simulink model "sistema (1)"  (R2025b)
settings: Solver=ode23t  StartTime=0.0  StopTime=10.0  MaxStep=1e-3  RelTol=1e-3
libraries: slpidlib x1, simulink x1
settings DataIOCC: ReturnWorkspaceOutputs=off  TimeSaveName=t
settings DebuggingCC: AlgebraicLoopMsg=none  ArtificialAlgebraicLoopMsg=none  MaxConsecutiveZCsMsg=none

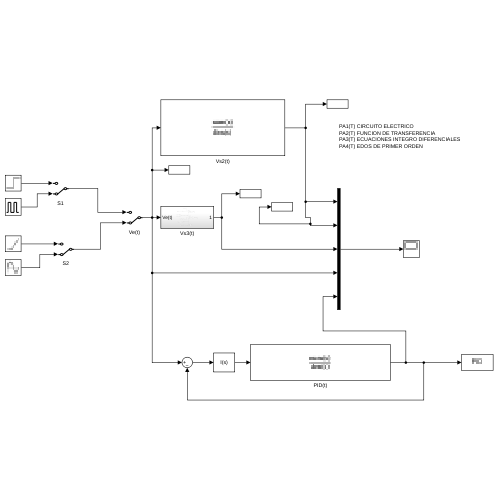
[thumbnail: Simulink's stored preview of the top-level diagram]
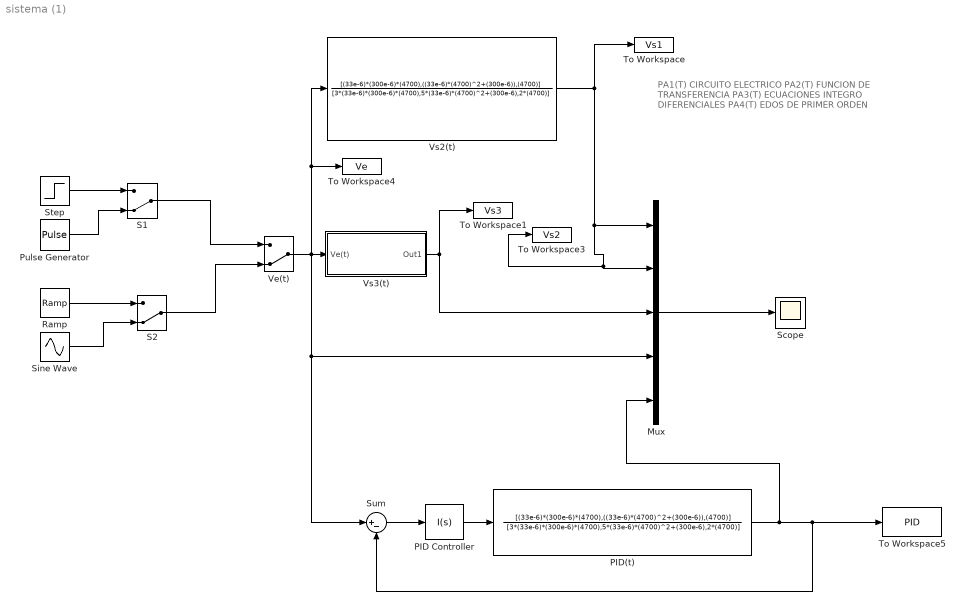
== system sistema (1) ==
  note: PA1(T) CIRCUITO ELECTRICO
      | PA2(T) FUNCION DE TRANSFERENCIA
      | PA3(T) ECUACIONES INTEGRO DIFERENCIALES
      | PA4(T) EDOS DE PRIMER ORDEN
  Mux : Mux  Inputs=5
  PID Controller : slpidlib/PID Controller  Controller=I  Form=Parallel  TimeDomain=Continuous-time  UseExternalTs=off  SampleTime=-1  IntegratorMethod=Forward Euler  FilterMethod=Forward Euler  ControllerParametersSource=internal  P=1  I=586.28935668378  UseKiTs=off  D=1  UseExternalDerivativeSource=off  N=1  UseFilter=on  TunerSelectOption=Transfer Function Based (PID Tuner App)  InitialConditionSource=internal  InitialConditionForIntegrator=0  InitialConditionForFilter=0  DifferentiatorICPrevScaledInput=0  ExternalReset=none  TrackingMode=off  Kt=1  LimitOutput=off  SatLimitsSource=internal  UpperSaturationLimit=inf  LowerSaturationLimit=-inf  LinearizeAsGain=on  AntiWindupMode=none  Kb=1  LimitIntegrator=off  UpperIntegratorSaturationLimit=inf  LowerIntegratorSaturationLimit=-inf  POutMin=[]  POutMax=[]  IOutMin=[]  IOutMax=[]  DOutMin=[]  DOutMax=[]  NOutMin=[]  NOutMax=[]  SumOutMin=[]  SumOutMax=[]  SaturationOutMin=[]  SaturationOutMax=[]  PParamMin=[]  PParamMax=[]  IParamMin=[]  IParamMax=[]  DParamMin=[]  DParamMax=[]  NParamMin=[]  NParamMax=[]  KbParamMin=[]  KbParamMax=[]  KtParamMin=[]  KtParamMax=[]  KbOutMin=[]  KbOutMax=[]  KtOutMin=[]  KtOutMax=[]  IntegratorOutMin=[]  IntegratorOutMax=[]  FilterOutMin=[]  FilterOutMax=[]  SumI1OutMin=[]  SumI1OutMax=[]  SumI2OutMin=[]  SumI2OutMax=[]  SumI3OutMin=[]  SumI3OutMax=[]  SumI4OutMin=[]  SumI4OutMax=[]  SumDOutMin=[]  SumDOutMax=[]  DifferentiatorOutMin=[]  DifferentiatorOutMax=[]  FilterDiffOutCoefMin=[]  FilterDiffOutCoefMax=[]  ReciprocalOutMin=[]  ReciprocalOutMax=[]  SumDenOutMin=[]  SumDenOutMax=[]  SumNumOutMin=[]  SumNumOutMax=[]  DivideOutMin=[]  DivideOutMax=[]  UdiffTsProdOutMin=[]  UdiffTsProdOutMax=[]  NTsProdOutMin=[]  NTsProdOutMax=[]  UintegralTsProdOutMin=[]  UintegralTsProdOutMax=[]  UngainTsProdOutMin=[]  UngainTsProdOutMax=[]  ClampingZeroOutDataTypeStr=Inherit: Inherit via back propagation  ClampingZeroOutMin=[]  ClampingZeroOutMax=[]  FilterDenConstantOutDataTypeStr=Inherit: Inherit via back propagation  FilterDenConstantOutMin=[]  FilterDenConstantOutMax=[]  PCopyOutDataTypeStr=Inherit: Inherit via back propagation  PCopyOutMin=[]  PCopyOutMax=[]  NCopyOutDataTypeStr=Inherit: Inherit via back propagation  NCopyOutMin=[]  NCopyOutMax=[]  IntegratorContinuousStateAttributes=''  IntegratorStateMustResolveToSignalObject=off  IntegratorRTWStateStorageClass=Auto  FilterContinuousStateAttributes=''  FilterStateMustResolveToSignalObject=off  FilterRTWStateStorageClass=Auto  ParallelPVariant=Disabled  IdealPVariant=Disabled  IVariant=InternalParameters  DVariant=Disabled  IntegratorVariant=Continuous  SatVariant=Disabled  AWVariant=Passthrough  PCopyVariant=Disabled  TRVariant=Disabled  FdbkBlocksVariant=Forward  IdealPFdbkVariant=Disabled  SatFdbkVariant=Disabled  DerivativeFilterVariant=Disabled  NVariant=Disabled  NCopyVariant=Disabled_SignalSpec  FilterICVariant=Disabled  IntegratorICVariant=InternalICs  ExternalResetVariant=Disabled  TRSumVariant=Passthrough  SumFdbkVariant=Disabled  SumVariant=Passthrough_I  TsampFilterVariant=InternalTs  TsampNgainVariant=Passthrough  TsampIntegralVariant=Disabled_SignalSpec  ExternalSaturationOutDataTypeStr=Inherit: Same as second input  DerivativeSourceVariant=Disabled  PreIntVariant=InternalPreInt
  PID(t) : TransferFcn  Numerator=[(33e-6)*(300e-6)*(4700),((33e-6)*(4700)^2+(300e-6)),(4700)]  Denominator=[3*(33e-6)*(300e-6)*(4700),5*(33e-6)*(4700)^2+(300e-6),2*(4700)]
  Pulse Generator : DiscretePulseGenerator  PulseType=Time based  Period=10  PulseWidth=10  PhaseDelay=1
  Ramp : simulink/Sources/Ramp  slope=1/10  start=0  InitialOutput=0
  S1 : ManualSwitch  CurrentSetting=0
  S2 : ManualSwitch  CurrentSetting=0
  Scope : Scope
      settings: ActiveDisplayYMinimum=-1.8078345673830822  ActiveDisplayYMaximum=1.5764968800691457
  Sine Wave : Sin  Frequency=pi/2  SampleTime=0
  Step : Step  Time=0  SampleTime=0.001
  Sum : Sum  Inputs=|+-
  To Workspace : ToWorkspace  VariableName=Vs1  SampleTime=-1
  To Workspace1 : ToWorkspace  VariableName=Vs3  SampleTime=-1
  To Workspace3 : ToWorkspace  VariableName=Vs2  SampleTime=-1
  To Workspace4 : ToWorkspace  VariableName=Ve  SampleTime=-1
  To Workspace5 : ToWorkspace  VariableName=PID  SampleTime=-1
  Ve(t) : ManualSwitch  CurrentSetting=0
  Vs2(t) : TransferFcn  Numerator=[(33e-6)*(300e-6)*(4700),((33e-6)*(4700)^2+(300e-6)),(4700)]  Denominator=[3*(33e-6)*(300e-6)*(4700),5*(33e-6)*(4700)^2+(300e-6),2*(4700)]
  Vs3(t) : Subsystem
  wires:
  Step/1 -> S1/1
  Pulse Generator/1 -> S1/2
  Ramp/1 -> S2/1
  Sine Wave/1 -> S2/2
  S1/1 -> Ve(t)/1
  S2/1 -> Ve(t)/2
  Ve(t)/1 -> Sum/1, Mux/4, To Workspace4/1, Vs2(t)/1, Vs3(t)/1(Ve(t))
  Vs2(t)/1 -> To Workspace/1, To Workspace3/1, Mux/2, Mux/1
  Vs3(t)/1(Out1) -> To Workspace1/1, Mux/3
  Mux/1 -> Scope/1
  Sum/1 -> PID Controller/1
  PID Controller/1 -> PID(t)/1
  PID(t)/1 -> Mux/5, To Workspace5/1, Sum/2

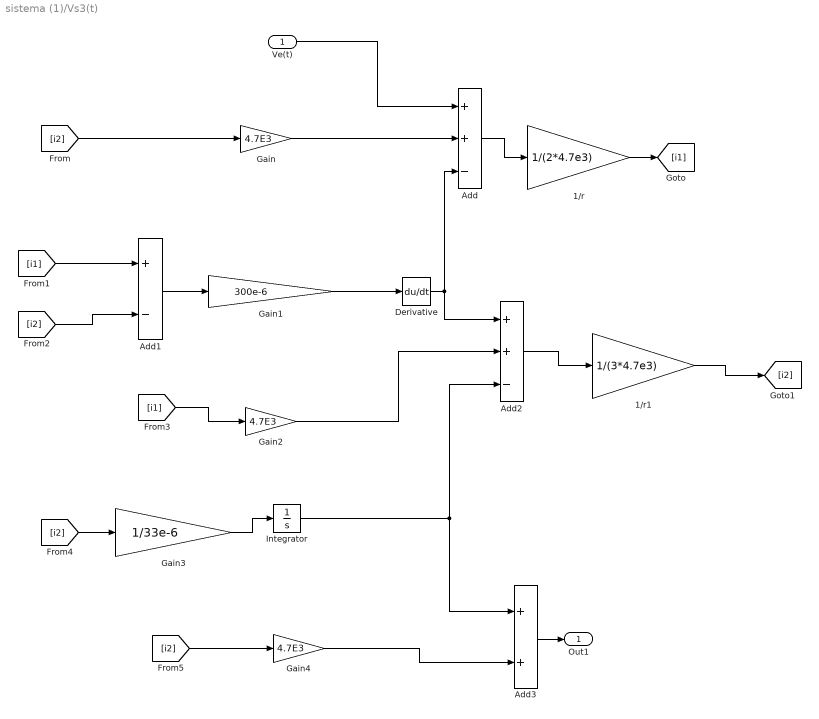
== system sistema (1)/Vs3(t) ==
  Ve(t) : Inport
  1/r : Gain  Gain=1/(2*4.7e3)
  1/r1 : Gain  Gain=1/(3*4.7e3)
  Add : Sum  Inputs=++-
  Add1 : Sum  Inputs=+-
  Add2 : Sum  Inputs=++-
  Add3 : Sum
  Derivative : Derivative
  Gain : Gain  Gain=4.7E3
  Gain1 : Gain  Gain=300e-6
  Gain2 : Gain  Gain=4.7E3
  Gain3 : Gain  Gain=1/33e-6
  Gain4 : Gain  Gain=4.7E3
  Integrator : Integrator
  Out1 : Outport
  wires:
  Add/1 -> 1/r/1
  Ve(t)/1 -> Add/1
  1/r/1 -> [i1]
  [i2] -> Gain/1
  Gain/1 -> Add/2
  [i1] -> Add1/1
  [i2] -> Add1/2
  Add1/1 -> Gain1/1
  Gain1/1 -> Derivative/1
  Derivative/1 -> Add/3, Add2/1
  [i1] -> Gain2/1
  Gain2/1 -> Add2/2
  [i2] -> Gain3/1
  Gain3/1 -> Integrator/1
  Integrator/1 -> Add3/1, Add2/3
  [i2] -> Gain4/1
  Gain4/1 -> Add3/2
  Add3/1 -> Out1/1
  Add2/1 -> 1/r1/1
  1/r1/1 -> [i2]
